simulink model "x2_observer"  (R2023b)
settings: Solver=VariableStepAuto  StartTime=0.0  StopTime=5.0  RelTol=1e-6
undefined symbols (not defined in the file): A, B, C, K, L, x1_e, x2_e
settings Model: Creator=adamo  LastModifiedBy=beniaminosquitieri

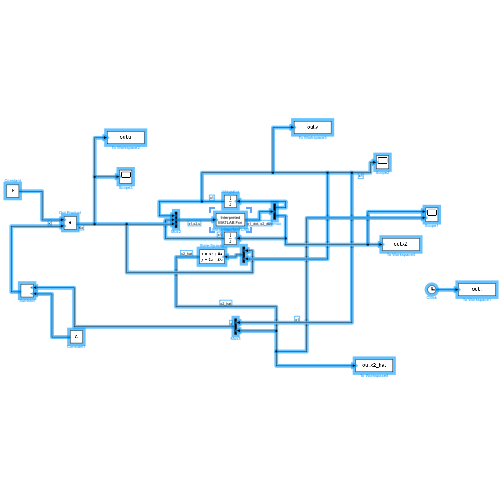
[thumbnail: Simulink's stored preview of the top-level diagram]
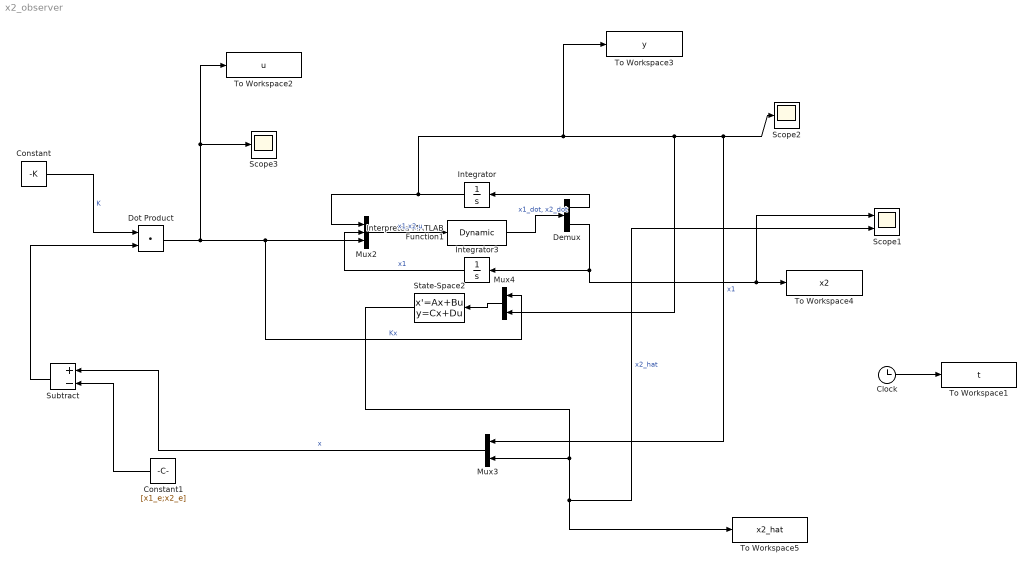
== system x2_observer ==
  Clock : Clock
  Constant : Constant  Value=-K
  Constant1 : Constant  Value=[x1_e;x2_e]
  Demux : Demux  Outputs=2
  Dot Product : DotProduct  OutDataTypeStr=Inherit: Inherit via internal rule
  Integrator : Integrator
  Integrator3 : Integrator
  Interpreted MATLAB Function1 : MATLABFcn  MATLABFcn=Dynamic  OutputDimensions=2
  Mux2 : Mux  Inputs=3
  Mux3 : Mux  Inputs=2
  Mux4 : Mux  Inputs=2
  Scope1 : Scope  NumInputPorts=2
  Scope2 : Scope
  Scope3 : Scope
  State-Space2 : StateSpace  A=A-L*C  B=[B L]  C=[0 1]  D=[0 0]  InitialCondition=[0 0]
  Subtract : Sum  Inputs=+-
  To Workspace1 : ToWorkspace  VariableName=t  SampleTime=-1
  To Workspace2 : ToWorkspace  VariableName=u  SampleTime=-1
  To Workspace3 : ToWorkspace  VariableName=y  SampleTime=-1
  To Workspace4 : ToWorkspace  VariableName=x2  SampleTime=-1
  To Workspace5 : ToWorkspace  VariableName=x2_hat  SampleTime=-1
  wires:
  Constant1/1 -> Subtract/2
  Constant/1 -> Dot Product/1  "K"
  Demux/2 -> Scope1/1, To Workspace4/1, Integrator3/1
  Integrator/1 -> To Workspace3/1, Mux4/2, Mux3/1, Scope2/1, Mux2/1  "x1"
  Integrator3/1 -> Mux2/2  "x1"
  Demux/1 -> Integrator/1
  Clock/1 -> To Workspace1/1
  Mux2/1 -> Interpreted MATLAB Function1/1  "x1,x2,u"
  Mux4/1 -> State-Space2/1
  Dot Product/1 -> To Workspace2/1, Scope3/1, Mux4/1, Mux2/3  "Kx"
  Interpreted MATLAB Function1/1 -> Demux/1  "x1_dot, x2_dot"
  State-Space2/1 -> Scope1/2, To Workspace5/1, Mux3/2  "x2_hat"
  Subtract/1 -> Dot Product/2
  Mux3/1 -> Subtract/1  "x"
